simulink model "first_astatism_system"  (R2021b)
settings: Solver=VariableStepAuto  StartTime=0.0  StopTime=10.0  RelTol=1e-3
settings Model: Creator=den  LastModifiedBy=den

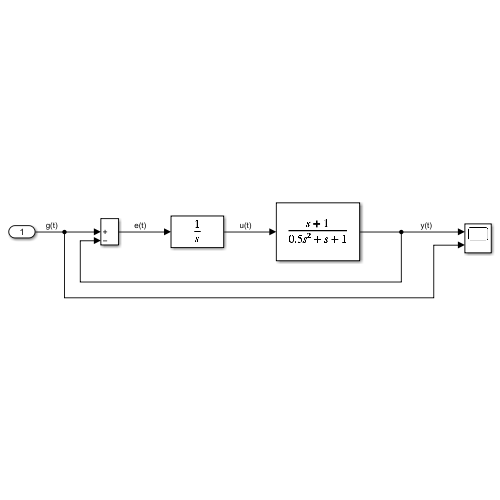
[thumbnail: Simulink's stored preview of the top-level diagram]
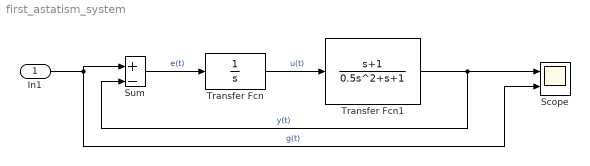
== system first_astatism_system ==
  In1 : Inport
  Scope : Scope  NumInputPorts=2
  Sum : Sum  Inputs=|+-
  Transfer Fcn : TransferFcn  Denominator=[1 0]
  Transfer Fcn1 : TransferFcn  Numerator=[1 1]  Denominator=[0.5 1 1]
  wires:
  Transfer Fcn/1 -> Transfer Fcn1/1  "u(t)"
  Transfer Fcn1/1 -> Sum/2, Scope/1  "y(t)"
  In1/1 -> Scope/2, Sum/1  "g(t)"
  Sum/1 -> Transfer Fcn/1  "e(t)"
